simulink model "synchroreelle"  (R2020b)
settings: Solver=FixedStepDiscrete  StartTime=0.0  StopTime=10  RelTol=1e-3
undefined symbols (not defined in the file or in its folder): j
libraries: simulink x1, dspstat3 x1, commsdrhw_v2 x1, dspsigops x1
Description:
  | This model uses Universal Software Radio Peripheral (USRP) hardware with Simulink(R) to perform FM demodulation and stereo decoding.
settings Model: Creator=druffle  LastModifiedBy=druffle
settings DataIOCC: SaveFormat=Structure  SaveOutput=off  SignalLogging=off  DSMLogging=off  SaveTime=off  ReturnWorkspaceOutputs=off
settings OptimizationCC: ExpressionDepthLimit=2147483647  EfficientMapNaN2IntZero=off  LifeSpan=inf  SimCompilerOptimization=on
settings DebuggingCC: UnderspecifiedInitializationDetection=Classic  MergeDetectMultiDrivingBlocksExec=none  SolverPrmCheckMsg=warning  InheritedTsInSrcMsg=none  MultiTaskCondExecSysMsg=none  ParameterPrecisionLossMsg=none  FcnCallInpInsideContextMsg=warning  AllowSymbolicDim=off  StateNameClashWarn=warning  SFUnexpectedBacktrackingDiag=warning  SFNoUnconditionalDefaultTransitionDiag=warning  SFExecutionAtInitializationDiag=none  ArithmeticOperatorsInVariantConditions=warning
settings HardwareCC: ProdBitPerPointer=32  ProdBitPerSizeT=32  ProdBitPerPtrDiffT=32  ProdLargestAtomicFloat=None  ProdIntDivRoundTo=Undefined  ProdEndianess=Unspecified  ProdWordSize=32  ProdHWDeviceType=32-bit Generic  TargetBitPerPointer=64  TargetBitPerSizeT=64  TargetBitPerPtrDiffT=64  TargetLongLongMode=on  TargetIntDivRoundTo=Zero  TargetEndianess=LittleEndian  TargetWordSize=64  TargetHWDeviceType=Generic->MATLAB Host Computer  ProdEqTarget=off
settings ModelReferenceCC: PropagateSignalLabelsOutOfModel=off
settings SFSimCC: SimIntegrity=off  SimUseLocalCustomCode=off  CustomCodeUndefinedFunction=UseInterfaceOnly
settings RTWCC: RTWUseLocalCustomCode=off
settings RTWCC: CustomSourceCode=|
  | #include <stdio.h>
  | #include <stdlib.h>
settings CodeAppCC: MaxIdLength=128  StateflowObjectComments=on
settings GRTTargetCC: TargetLangStandard=C89/C90 (ANSI)  CombineOutputUpdateFcns=off  GRTInterface=on
settings ConfigComp: CovMetricSettings=dw  CovSaveCumulativeToWorkspaceVar=on  CovSaveSingleToWorkspaceVar=on  CovExternalEMLEnable=off  CovSFcnEnable=off

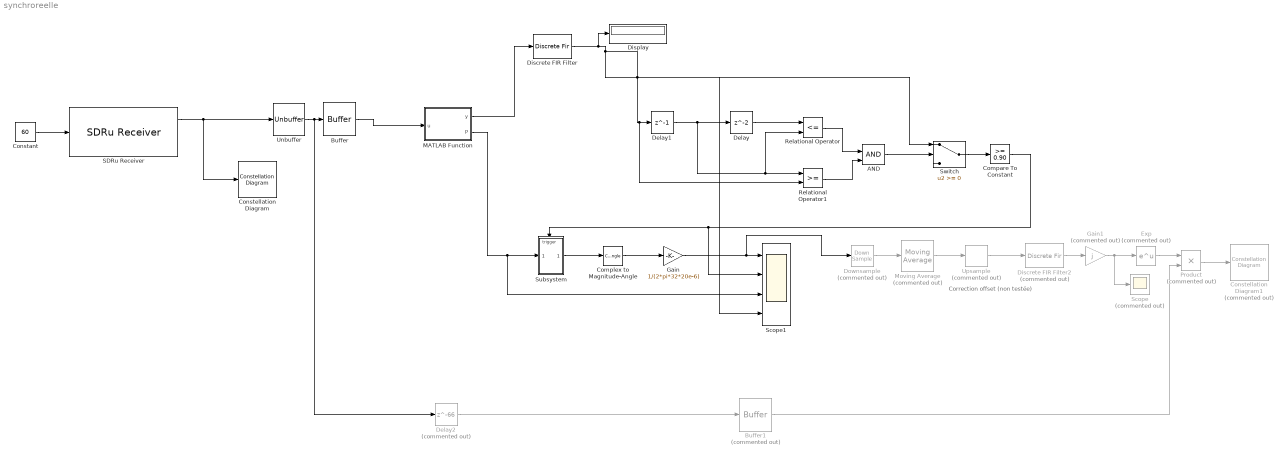
== system synchroreelle ==
  note: Correction offset (non testée)
  AND : Logic  IconShape=distinctive  AllPortsSameDT=off  OutDataTypeStr=boolean
  Buffer : Buffer  V=63  OutputFrames=off
  Buffer1 : Buffer  Commented=on  N=660  OutputFrames=off
  Compare To Constant : simulink/Logic and Bit Operations/Compare To Constant  relop=>=  const=0.90  OutDataTypeStr=boolean
  Complex to Magnitude-Angle : ComplexToMagnitudeAngle  Output=Angle
  Constant : Constant  Value=60
  Constellation Diagram : ConstellationDiagram
  Constellation Diagram1 : ConstellationDiagram  Commented=on
  Delay : Delay
  Delay1 : Delay  DelayLength=1
  Delay2 : Delay  Commented=on  DelayLength=66
  Discrete FIR Filter : DiscreteFir  Coefficients=[1/3 1/3 1/3]
  Discrete FIR Filter2 : DiscreteFir  Commented=on  Coefficients=[ones(660, 1)]
  Display : Display
  Downsample : DownSample  Commented=on  N=660
  Exp : Math  Commented=on  OutputSignalType=complex  SaturateOnIntegerOverflow=on
  Gain : Gain  Gain=1/(2*pi*32*20e-6)
  Gain1 : Gain  Commented=on  Gain=j
  MATLAB Function : MATLAB Function  TreatAsAtomicUnit=on
  Moving Average : dspstat3/Moving Average  Commented=on  Method=Sliding window  ForgettingFactorPort=off  SpecifyWindowLength=on  WindowLength=50  ForgettingFactor=0.9  SimulateUsing=Code generation
  Product : Product  Commented=on
  Relational Operator : RelationalOperator  Operator=<=  OutDataTypeStr=boolean  RndMeth=Simplest
  Relational Operator1 : RelationalOperator  OutDataTypeStr=boolean  RndMeth=Simplest
  SDRu Receiver : commsdrhw_v2/SDRu Receiver  rxtx=rx  initializeIPAddress=0  devMap=10  USRP2_IP=192.168.10.2  USRP_IP_X300=192.168.10.2  USRP_IP_X310=No devices found  USRP_IP_N300=192.168.10.2  USRP_IP_N310=192.168.10.2  USRP_IP_N320=192.168.10.2  USRP_serialNumB200=No devices found  USRP_serialNumB210=30CEEA7  platform=B210  prevPlatform=B210  lastIPAddressPopup=192.168.10.2  USRP_ID=30CEEA7  LastIPAddress=192.168.10.2  IsTwinRXDaughterboard=off  EnableTwinRXPhaseSync=off  losrc=0  ChannelMapping=1  centerFrequencySrc=Dialog  centerFrequency=433e6  loOffsetSrc=Dialog  loOffset=0  gainSrc=Input port  gain=60  PPSSource=Internal  clockSource=Internal  masterClkRateParam=25600000  masterClkRateB200=32e6  masterClkRateB210=25.6e6  masterClkRateX300=200e6  masterClkRateX310=200e6  masterClkRateN300=125e6  masterClkRateN310=125e6  masterClkRateN320=200e6  masterClkRate=100e6  masterClkRateTwinRX=200e6  decimInterpSrc=Dialog  decimInterpPort=512  lastDecimSource=Dialog  decimInterp=512  USRP2_IP_NUM=[51 48 67 69 69 65 55]  sampleRate=50000  sampleTime=512/25600000  TransportDataType=int16  overrunUnderrunPort=off  outputDatatype=double  frameLength=660  HOST_DATA_PORT=0  HOST_CONTROL_PORT=0  USRP2_DATA_PORT=0  USRP2_CONTROL_PORT=0  bufferMode=Continuous streaming  EnableBurstMode=on  NumFramesInBurst=10
      settings: SourceProductBaseCode=USRP
  Scope : Scope  Commented=on
  Scope1 : Scope  NumInputPorts=4
  Subsystem : Subsystem
  Switch : Switch
  Unbuffer : Unbuffer
  Upsample : dspsigops/Upsample  Commented=on  N=660  phase=0  RateOptions=Allow multirate processing  ic=0  mode=Unused parameter value
  wires:
  Switch/1 -> Compare To Constant/1
  Relational Operator1/1 -> AND/2
  MATLAB Function/1(y) -> Discrete FIR Filter/1
  AND/1 -> Switch/2
  Compare To Constant/1 -> Subsystem/Trigger, Scope1/2
  Delay1/1 -> Relational Operator/2, Relational Operator1/1, Delay/1
  Buffer/1 -> MATLAB Function/1(u)
  Subsystem/1(Out1) -> Complex to Magnitude-Angle/1
  Relational Operator/1 -> AND/1
  MATLAB Function/2(P) -> Scope1/3, Subsystem/1(In1)
  Discrete FIR Filter/1 -> Display/1, Scope1/4, Switch/1, Relational Operator1/2, Delay1/1
  Delay/1 -> Relational Operator/1
  Gain/1 -> Downsample/1, Scope1/1
  Complex to Magnitude-Angle/1 -> Gain/1
  Unbuffer/1 -> Delay2/1, Buffer/1
  Constant/1 -> SDRu Receiver/1
  Upsample/1 -> Discrete FIR Filter2/1
  Downsample/1 -> Moving Average/1
  Moving Average/1 -> Upsample/1
  Discrete FIR Filter2/1 -> Gain1/1
  Exp/1 -> Product/1
  Product/1 -> Constellation Diagram1/1
  SDRu Receiver/1 -> Constellation Diagram/1, Unbuffer/1
  Buffer1/1 -> Product/2
  Delay2/1 -> Buffer1/1
  Gain1/1 -> Exp/1, Scope/1

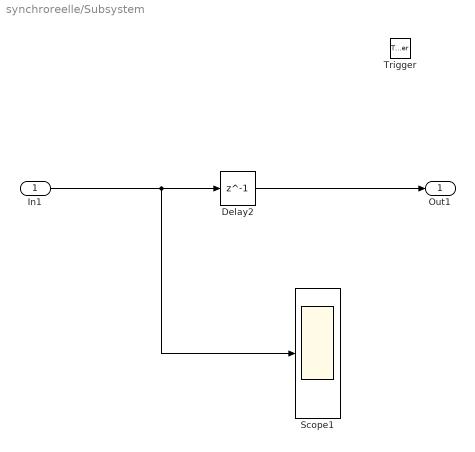
== system synchroreelle/Subsystem ==
  In1 : Inport
  Trigger : TriggerPort  VariantControl=Variant  PortDimensions=1
  Delay2 : Delay  DelayLength=1
  Scope1 : Scope
  Out1 : Outport
  wires:
  In1/1 -> Scope1/1, Delay2/1
  Delay2/1 -> Out1/1

== matlab function synchroreelle/MATLAB Function ==
  data: u input; y output; P output
function [y, P]= fcn(u)

    L = 32;

    samples = u;
    t = length(samples);
    T = 64*20e-6;
    start = 1;
    Ng = 3;
    ds = 1;
    d=0;

    % Initialiser à zéro
    %phi = zeros(1, uint64((t/(2*L))+1));
    %res=zeros(1, uint64((t/(2*L))+1));
        % calculer la corrélation entre les échantillons d et d+L
        P = sum(samples(d+L+1:d+L+L) .* conj(samples(d+1:d+L)));
        % normaliser la corrélation par l'énergie du demi-symbole
        R = sum(abs(samples(d+1+L:d+L+L)).^2);
        Rf=(1/2)*(sum(abs(samples(d:d+63).^2)));
        % vérifier que corr et energy ne sont pas égaux à zéro
        if P ~= 0 && R ~= 0
            M = abs(P).^2 ./ R.^2;
        else
            M = 0;
        end
        if P~=0 && Rf ~=0
             Mf = abs(P).^2 ./ Rf.^2;
        else
             Mf = 0;
        end

   
       
    


    

y = Mf;
